simulink model "newtons_cooling_law"  (R2022a)
settings: Solver=VariableStepAuto  StartTime=0.0  StopTime=100  RelTol=1e-3
settings Model: Creator=Home computer  LastModifiedBy=Home computer

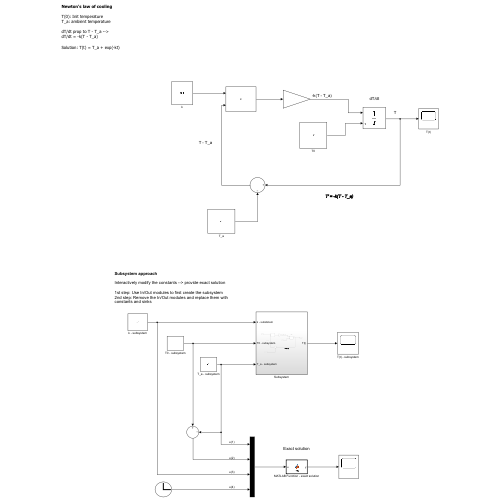
[thumbnail: Simulink's stored preview of the top-level diagram]
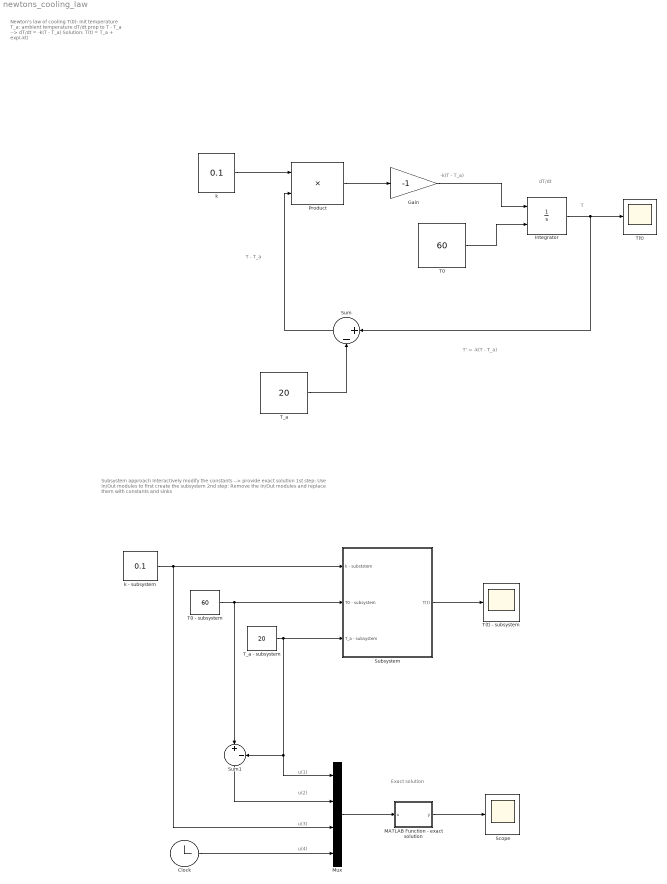
== system newtons_cooling_law ==
  note: Exact solution
  note: u(1)
  note: u(2)
  note: u(4)
  note: u(3)
  note: Subsystem approach
      |
      | Interactively modify the constants --> provide exact solution
      |
      | 1st step: Use In/Out modules to first create the subsystem
      | 2nd step: Remove the In/Out modules and replace them with constants and sinks
  note: T - T_a
  note: -k(T - T_a)
  note: T' = -k(T - T_a)
  note: T
  note: dT/dt
  note: Newton's law of cooling
      |
      | T(0): Init temperature
      | T_a: ambient temperature
      |
      | dT/dt prop to T - T_a -->
      | dT/dt = -k(T - T_a)
      |
      | Solution: T(t) = T_a + exp(-kt)
  Clock : Clock
  Gain : Gain  Gain=-1
  Integrator : Integrator  InitialConditionSource=external
  MATLAB Function - exact solution : MATLAB Function  TreatAsAtomicUnit=on
  Mux : Mux
  Product : Product
  Scope : Scope
  Subsystem : Subsystem
  Sum : Sum  Inputs=|+-
  Sum1 : Sum  Inputs=|+-
  T(t) : Scope
  T(t) - subsystem : Scope
  T0 : Constant  Value=60
  T0 - subsystem : Constant  Value=60
  T_a : Constant  Value=20
  T_a - subsystem : Constant  Value=20
  k : Constant  Value=0.1
  k - subsystem : Constant  Value=0.1
  wires:
  k/1 -> Product/1
  Product/1 -> Gain/1
  Gain/1 -> Integrator/1
  Integrator/1 -> Sum/1, T(t)/1
  T0/1 -> Integrator/2
  T_a/1 -> Sum/2
  Sum/1 -> Product/2
  k - subsystem/1 -> Mux/3, Subsystem/1(k - subststem)
  T0 - subsystem/1 -> Subsystem/2(T0 - subsystem), Sum1/1
  T_a - subsystem/1 -> Subsystem/3(T_a - subsystem), Mux/1, Sum1/2
  Subsystem/1(T(t)) -> T(t) - subsystem/1
  Mux/1 -> MATLAB Function - exact solution/1(u)
  Clock/1 -> Mux/4
  Sum1/1 -> Mux/2
  MATLAB Function - exact solution/1(y) -> Scope/1

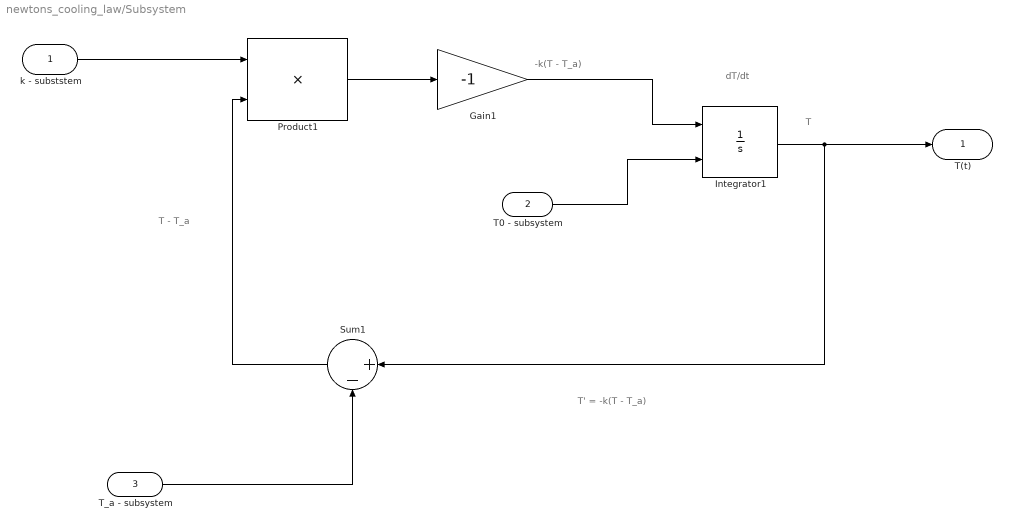
== system newtons_cooling_law/Subsystem ==
  note: T - T_a
  note: T' = -k(T - T_a)
  note: dT/dt
  note: T
  note: -k(T - T_a)
  k - subststem : Inport
  T0 - subsystem : Inport  Port=2
  T_a - subsystem : Inport  Port=3
  Gain1 : Gain  Gain=-1
  Integrator1 : Integrator  InitialConditionSource=external
  Product1 : Product
  Sum1 : Sum  Inputs=|+-
  T(t) : Outport
  wires:
  T0 - subsystem/1 -> Integrator1/2
  Gain1/1 -> Integrator1/1
  Integrator1/1 -> T(t)/1, Sum1/1
  Sum1/1 -> Product1/2
  k - subststem/1 -> Product1/1
  Product1/1 -> Gain1/1
  T_a - subsystem/1 -> Sum1/2

== matlab function newtons_cooling_law/MATLAB Function - exact solution ==
  data: u input; y output
function y = fcn(u)

% u(1): T_a
% u(2): T0 - T_a
% u(3): k
% u(4): t
y = u(1)+u(2)*exp(-u(3)*u(4));
